simulink model "program_simulink_3"  (R2024b)
settings: Solver=VariableStepAuto  StartTime=0.0  StopTime=13  RelTol=1e-3
undefined symbols (not defined in the file): magnitude
settings Model: Creator=俞书阳  LastModifiedBy=user

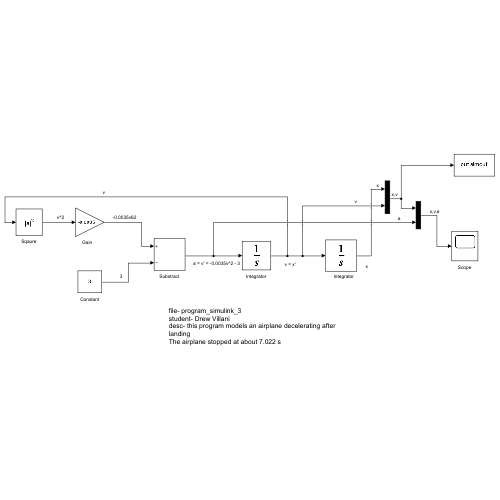
[thumbnail: Simulink's stored preview of the top-level diagram]
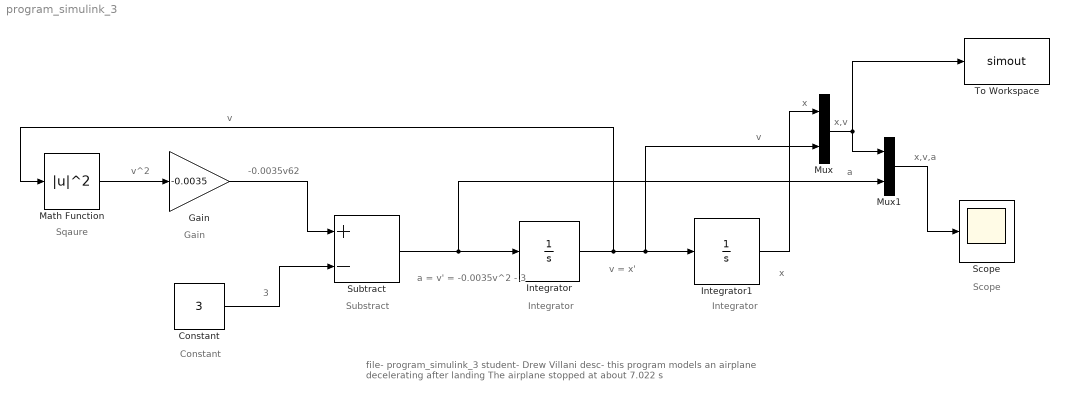
== system program_simulink_3 ==
  note: file- program_simulink_3
      | student- Drew Villani
      | desc- this program models an airplane decelerating after landing
      | The airplane stopped at about 7.022 s
  note: -0.0035v62
  note: v^2
  note: v
  note: a = v' = -0.0035v^2 - 3
  note: x
  note: v
  note: a
  note: x,v
  note: x,v,a
  note: x
  note: v = x'
  note: 3
  note: Scope
  note: Integrator
  note: Gain
  note: Sqaure
  note: Substract
  note: Constant
  note: Integrator
  Constant : Constant  Value=3
  Gain : Gain  Gain=-0.0035
  Integrator : Integrator
  Integrator1 : Integrator  InitialCondition=83.33
  Math Function : Math  Operator=magnitude^2
  Mux : Mux  Inputs=2
  Mux1 : Mux  Inputs=2
  Scope : Scope
  Subtract : Sum  Inputs=+-
  To Workspace : ToWorkspace  VariableName=simout  SaveFormat=Timeseries  SampleTime=-1
  wires:
  Constant/1 -> Subtract/2
  Gain/1 -> Subtract/1
  Subtract/1 -> Mux1/2, Integrator/1
  Integrator/1 -> Mux/2, Integrator1/1, Math Function/1
  Math Function/1 -> Gain/1
  Integrator1/1 -> Mux/1
  Mux/1 -> To Workspace/1, Mux1/1
  Mux1/1 -> Scope/1
